simulink model "lab3_q"  (R2018a)
settings: Solver=VariableStepAuto  StartTime=0.0  StopTime=t_max  RelTol=1e-3
undefined symbols (not defined in the file): k, k2, Lo, Mo, t0, y0
settings Model: Creator=lev  LastModifiedBy=lev
settings DebuggingCC: LibraryContextMissingDiagnostic=warning
settings SFSimCC: SimUseLocalCustomCode=on
settings RTWCC: RTWUseLocalCustomCode=on

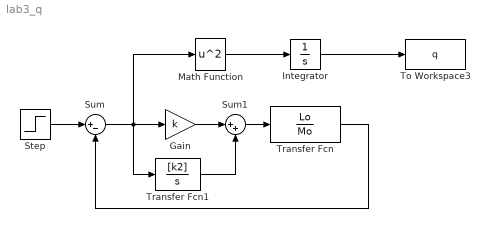
== system lab3_q ==
  Gain : Gain  Gain=k
  Integrator : Integrator
  Math Function : Math  Operator=square  SaturateOnIntegerOverflow=on
  Step : Step  Time=t0  After=y0  SampleTime=0
  Sum : Sum  Inputs=|+-
  Sum1 : Sum  Inputs=|++
  To Workspace3 : ToWorkspace  VariableName=q  SampleTime=-1
      settings: MaxDataPoints=1
  Transfer Fcn : TransferFcn  Numerator=Lo  Denominator=Mo
  Transfer Fcn1 : TransferFcn  Numerator=[k2]  Denominator=[1 0]
  wires:
  Transfer Fcn/1 -> Sum/2
  Sum/1 -> Math Function/1, Transfer Fcn1/1, Gain/1
  Step/1 -> Sum/1
  Sum1/1 -> Transfer Fcn/1
  Transfer Fcn1/1 -> Sum1/2
  Gain/1 -> Sum1/1
  Math Function/1 -> Integrator/1
  Integrator/1 -> To Workspace3/1
